simulink model "AFM_SS_linearFDBK_obs_trackCLQR"  (R2016b)
settings: Solver=VariableStepDiscrete  StartTime=0.0  StopTime=trun  FixedStep=Ts  EnableMultiTasking=on
undefined symbols (not defined in the file): absorbDelay, C_delay, Discrete, H, K_trk, Ki_trk, L, Nd_out, NoiseP, Ns, PLANT, swtch, sys_obs, Time, Ts, umax, X0_obs
libraries: cstblocks x2, simulink x1, powerlib_meascontrol x1, customLibFcns x1, ctrlSharedLib x1
settings Model: Creator=arnold  LastModifiedBy=arnold
settings DataIOCC: SaveFormat=Structure  SaveOutput=off  SaveState=on  InspectSignalLogs=on  TimeSaveName=tout_ptos
settings OptimizationCC: LifeSpan=inf
settings DebuggingCC: SolverPrmCheckMsg=warning  SFUnexpectedBacktrackingDiag=warning  SFNoUnconditionalDefaultTransitionDiag=warning  SFExecutionAtInitializationDiag=none
settings HardwareCC: ProdBitPerPointer=32  ProdBitPerSizeT=32  ProdBitPerPtrDiffT=32  ProdLargestAtomicFloat=None  ProdIntDivRoundTo=Undefined  ProdEndianess=Unspecified  ProdWordSize=32  ProdHWDeviceType=32-bit Generic
settings ModelReferenceCC: PropagateSignalLabelsOutOfModel=off
settings GRTTargetCC: TargetLangStandard=C89/C90 (ANSI)  GeneratePreprocessorConditionals=Disable all
settings ConfigComp: CovMetricSettings=dw  CovHtmlReporting=on  CovSaveCumulativeToWorkspaceVar=on  CovSaveSingleToWorkspaceVar=on  CovExternalEMLEnable=off  CovSFcnEnable=off

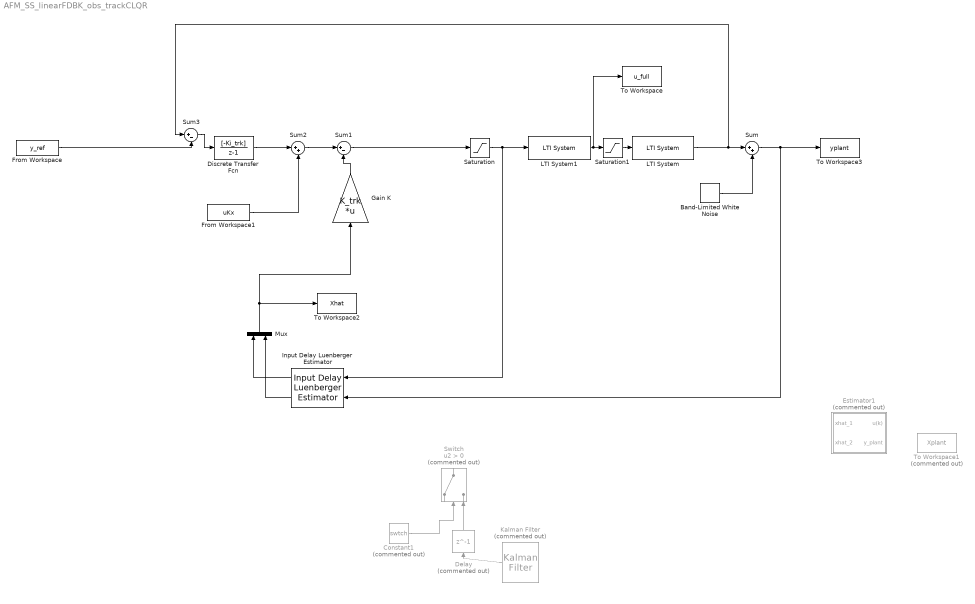
== system AFM_SS_linearFDBK_obs_trackCLQR ==
  Band-Limited White Noise : simulink/Sources/Band-Limited White Noise  Cov=[NoiseP]  Ts=Ts  seed=[23341]
  Constant1 : Constant  Commented=on  Value=swtch
  Delay : Delay  Commented=on  DelayLength=1
  Discrete Transfer Fcn : DiscreteTransferFcn  Numerator=[-Ki_trk]  Denominator=[1 -1]  SampleTime=Ts
  Estimator1 : Subsystem  Commented=on
  From Workspace : FromWorkspace  VariableName=y_ref  OutDataTypeStr=double  SampleTime=Ts
  From Workspace1 : FromWorkspace  VariableName=uKx  SampleTime=Ts
  Gain K : Gain  Gain=K_trk  Multiplication=Matrix(K*u)
  Input Delay Luenberger Estimator : customLibFcns/Input Delay Luenberger Estimator
      link override Delay4: InitialCondition=uss_0
      link override Discrete Shift Register: InitialValue=uss_0
  Kalman Filter : ctrlSharedLib/Kalman Filter  Commented=on  TimeDomain=Discrete-Time  UseCurrentEstimator=on  ModelSource=LTI State-Space Variable  ModelSourceVariable=sys_obsDesignK  A=0.95  B=1  C=1  D=0  NumberOfStates=1  NumberOfInputs=1  NumberOfOutputs=1  InitialEstimateSource=Dialog  X0=0  P0=10  UseK=off  UseGH=off  NumberOfProcessNoiseInputs=1  G=1  TimeInvariantG=on  H=0  TimeInvariantH=on  Q=0.05  TimeInvariantQ=on  R=1  TimeInvariantR=on  N=0  TimeInvariantN=on  AddInputPort=on  AddEnablePort=off  OutputEstimatedY=off  OutputP=off  Ts=-1
  LTI System : cstblocks/LTI System  sys=absorbDelay(PLANT)  IC=x0_full
  LTI System1 : cstblocks/LTI System  sys=g1_inv  IC=x0_full
  Mux : Mux  Inputs=2
  Saturation : Saturate  UpperLimit=umax  LowerLimit=-umax  OutDataTypeStr=double
  Saturation1 : Saturate  UpperLimit=umax  LowerLimit=-umax  OutDataTypeStr=double
  Sum : Sum  Inputs=|++
  Sum1 : Sum  Inputs=|+-
  Sum2 : Sum  Inputs=|++
  Sum3 : Sum  Inputs=|+-
  Switch : Switch  Commented=on  Criteria=u2 > Threshold
  To Workspace : ToWorkspace  VariableName=u_full  SaveFormat=Timeseries  SampleTime=Ts
      settings: Save2DSignal=2-D array (concatenate along first dimension)
  To Workspace1 : ToWorkspace  Commented=on  VariableName=Xplant  SaveFormat=Timeseries  SampleTime=-1
      settings: Save2DSignal=2-D array (concatenate along first dimension)
  To Workspace2 : ToWorkspace  VariableName=Xhat  SaveFormat=Timeseries  SampleTime=Ts
      settings: Save2DSignal=2-D array (concatenate along first dimension)
  To Workspace3 : ToWorkspace  VariableName=yplant  SaveFormat=Timeseries  SampleTime=Ts
      settings: Save2DSignal=2-D array (concatenate along first dimension)
  wires:
  LTI System/1 -> Sum/1, Sum3/1
  Gain K/1 -> Sum1/2
  Input Delay Luenberger Estimator/1 -> Mux/1
  Mux/1 -> To Workspace2/1, Gain K/1
  Constant1/1 -> Switch/2
  Input Delay Luenberger Estimator/2 -> Mux/2
  From Workspace/1 -> Sum3/2
  Sum3/1 -> Discrete Transfer Fcn/1
  Sum2/1 -> Sum1/1
  Kalman Filter/1 -> Delay/1
  Delay/1 -> Switch/3
  Sum/1 -> Input Delay Luenberger Estimator/2, To Workspace3/1
  Band-Limited White Noise/1 -> Sum/2
  Saturation/1 -> LTI System1/1, Input Delay Luenberger Estimator/1
  Sum1/1 -> Saturation/1
  From Workspace1/1 -> Sum2/2
  Discrete Transfer Fcn/1 -> Sum2/1
  LTI System1/1 -> To Workspace/1, Saturation1/1
  Saturation1/1 -> LTI System/1

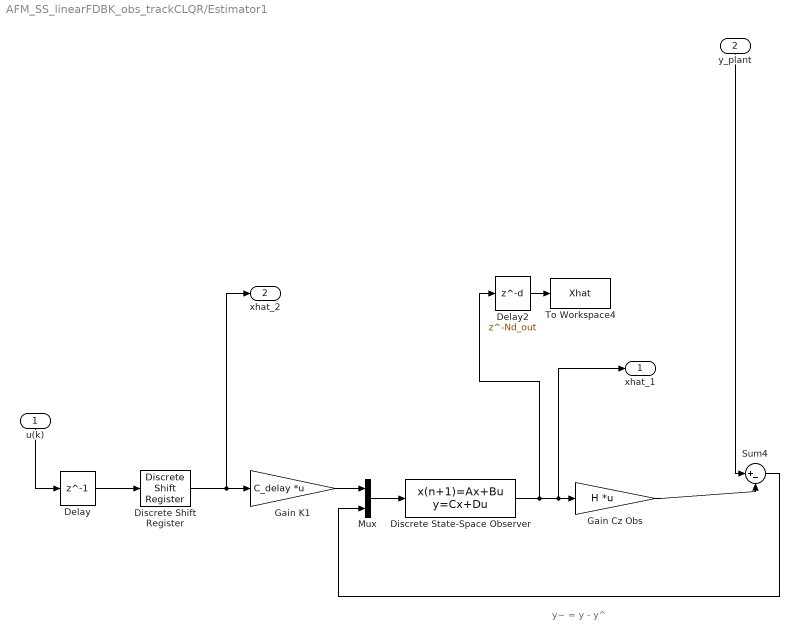
== system AFM_SS_linearFDBK_obs_trackCLQR/Estimator1 ==
  note: y~ = y - y^
  u(k) : Inport
  y_plant : Inport  Port=2
  Delay : Delay  DelayLength=1
  Delay2 : Delay  DelayLength=Nd_out
  Discrete Shift Register : powerlib_meascontrol/Additional Components/Discrete Shift Register  NSamples=Nd  InitialValue=0  Ts=Ts
  Discrete State-Space Observer : DiscreteStateSpace  A=sys_obs.a  B=[sys_obs.b, L]  C=eye(Ns)  D=zeros(Ns,2)  X0=X0_obs  SampleTime=Ts
  Gain Cz Obs : Gain  Gain=H  Multiplication=Matrix(K*u)
  Gain K1 : Gain  Gain=C_delay  Multiplication=Matrix(K*u)
  Mux : Mux  Inputs=2
  Sum4 : Sum  Inputs=|+-
  To Workspace4 : ToWorkspace  VariableName=Xhat  SaveFormat=Timeseries  SampleTime=-1
      settings: Save2DSignal=2-D array (concatenate along first dimension)
  xhat_1 : Outport
  xhat_2 : Outport  Port=2
  wires:
  Mux/1 -> Discrete State-Space Observer/1
  Sum4/1 -> Mux/2
  Discrete State-Space Observer/1 -> Delay2/1, Gain Cz Obs/1, xhat_1/1
  y_plant/1 -> Sum4/1
  Gain Cz Obs/1 -> Sum4/2
  Delay2/1 -> To Workspace4/1
  Discrete Shift Register/1 -> xhat_2/1, Gain K1/1
  Delay/1 -> Discrete Shift Register/1
  Gain K1/1 -> Mux/1
  u(k)/1 -> Delay/1
